simulink library "MFMdl1"  (Simulink 8.8)
settings: Solver=VariableStepAuto  StartTime=0.0  StopTime=10.0  RelTol=1e-3
libraries: simulink x1
settings Model: Creator=viett  LastModifiedBy=viett

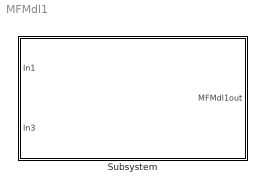
== system MFMdl1 ==
  Subsystem : Subsystem

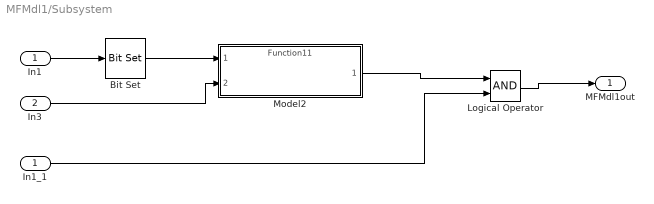
== system MFMdl1/Subsystem ==
  In1 : Inport
  In3 : Inport  Port=2
  Bit Set : simulink/Logic and Bit Operations/Bit Set  iBit=0
  In1_1 : InportShadow
  Logical Operator : Logic  AllPortsSameDT=off  OutDataTypeStr=boolean
  Model2 : ModelReference  ModelNameDialog=Function11.slx  SimulationMode=Normal  ModelReferenceVersion=1.20
  MFMdl1out : Outport
  wires:
  Logical Operator/1 -> MFMdl1out/1
  In1/1 -> Bit Set/1
  Bit Set/1 -> Model2/1
  Model2/1 -> Logical Operator/1
  In1_1/1 -> Logical Operator/2
  In3/1 -> Model2/2
